simulink model "exnb4137986_Q4"  (R2023b)
settings: Solver=FixedStepAuto  StartTime=0  StopTime=100  FixedStep=0.01  RelTol=1e-3
settings Model: Creator=therk  LastModifiedBy=therk

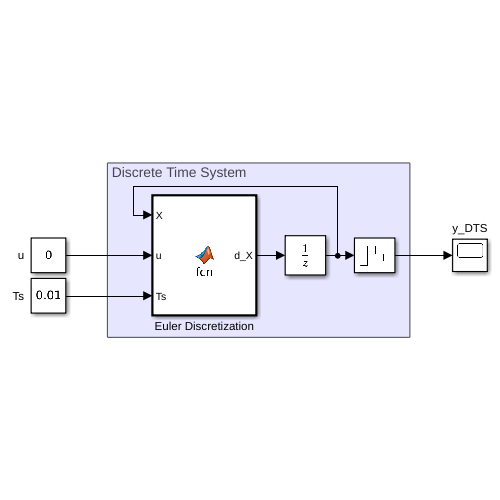
[thumbnail: Simulink's stored preview of the top-level diagram]
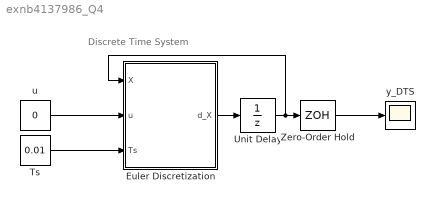
== system exnb4137986_Q4 ==
  note: Discrete Time System
  Euler Discretization : MATLAB Function  TreatAsAtomicUnit=on
  Ts : Constant  Value=0.01
  Unit Delay : UnitDelay  InitialCondition=[1;1]  SampleTime=-1  HasFrameUpgradeWarning=on
  Zero-Order Hold : ZeroOrderHold  SampleTime=-1
  u : Constant  Value=0
  y_DTS : Scope
  wires:
  Zero-Order Hold/1 -> y_DTS/1
  u/1 -> Euler Discretization/2(u)
  Unit Delay/1 -> Zero-Order Hold/1, Euler Discretization/1(X)
  Ts/1 -> Euler Discretization/3(Ts)
  Euler Discretization/1(d_X) -> Unit Delay/1

== matlab function exnb4137986_Q4/Euler Discretization ==
  data: X input; d_X output; u input; Ts input
function d_X = fcn(X, u, Ts)

Xdot = [X(1)*X(2)-X(1);
        -4/3*X(1)*X(2)+2/3*X(2)+u];

d_X = [X(1) + Ts*Xdot(1);
          X(2) + Ts*Xdot(2)];
